simulink model "StateSpace_Sim"  (R2018b)
settings: Solver=ode8  StartTime=0.0  StopTime=30  FixedStep=1/6  RelTol=1e-3
undefined symbols (not defined in the file): A, B, C, d_initial, K, L, M, x_initial, x_lin_i, x_soll
settings Model: Creator=Naresh  LastModifiedBy=Naresh

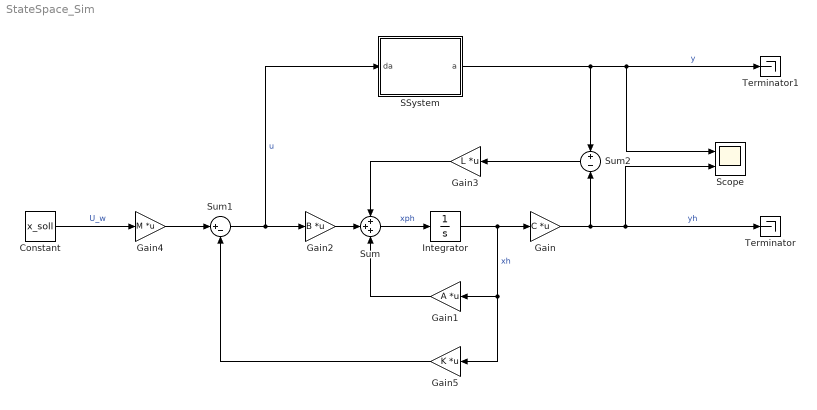
== system StateSpace_Sim ==
  Constant : Constant  Value=x_soll
  Gain : Gain  Gain=C  Multiplication=Matrix(K*u)
  Gain1 : Gain  Gain=A  Multiplication=Matrix(K*u)
  Gain2 : Gain  Gain=B  Multiplication=Matrix(K*u)
  Gain3 : Gain  Gain=L  Multiplication=Matrix(K*u)
  Gain4 : Gain  Gain=M  Multiplication=Matrix(K*u)
  Gain5 : Gain  Gain=K  Multiplication=Matrix(K*u)
  Integrator : Integrator  InitialCondition=x_lin_i
  SSystem : Subsystem
  Scope : Scope  NumInputPorts=2
  Sum : Sum  Inputs=+++
  Sum1 : Sum  Inputs=|+-
  Sum2 : Sum  Inputs=+|-
  Terminator : Terminator
  Terminator1 : Terminator
  wires:
  Integrator/1 -> Gain5/1, Gain1/1, Gain/1  "xh"
  Sum/1 -> Integrator/1  "xph"
  Sum1/1 -> SSystem/1(da), Gain2/1  "u"
  Gain4/1 -> Sum1/1
  Gain/1 -> Terminator/1, Scope/2, Sum2/2  "yh"
  SSystem/1(a) -> Sum2/1, Scope/1, Terminator1/1  "y"
  Sum2/1 -> Gain3/1
  Gain2/1 -> Sum/2
  Gain1/1 -> Sum/3
  Gain3/1 -> Sum/1
  Gain5/1 -> Sum1/2
  Constant/1 -> Gain4/1  "U_w"

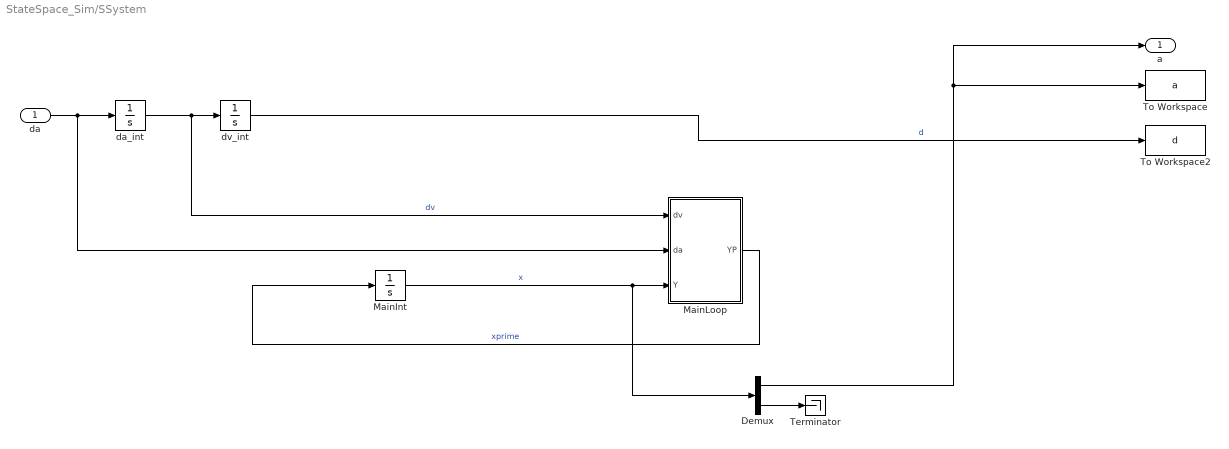
== system StateSpace_Sim/SSystem ==
  da : Inport
  Demux : Demux  Outputs=2
  MainInt : Integrator  InitialCondition=x_initial
  MainLoop : MATLAB Function  TreatAsAtomicUnit=on
  Terminator : Terminator
  To Workspace : ToWorkspace  VariableName=a  SaveFormat=Timeseries  SampleTime=-1
  To Workspace2 : ToWorkspace  VariableName=d  SaveFormat=Timeseries  SampleTime=-1
  da_int : Integrator  InitialCondition=d_initial(2)
  dv_int : Integrator  InitialCondition=d_initial(1)
  a : Outport
  wires:
  da/1 -> MainLoop/2(da), da_int/1
  MainInt/1 -> Demux/1, MainLoop/3(Y)  "x"
  da_int/1 -> MainLoop/1(dv), dv_int/1  "dv"
  MainLoop/1(YP) -> MainInt/1  "xprime"
  dv_int/1 -> To Workspace2/1  "d"
  Demux/2 -> Terminator/1
  Demux/1 -> a/1, To Workspace/1

== matlab function StateSpace_Sim/SSystem/MainLoop ==
  data: dv input; YP output; da input; Y input
function YP = MainLoop(dv,da,Y)
    g = 9.81;
    L = 10;
    m=2;
    lambda=1;

    YP = zeros(2,1);

    YP(1) = Y(2);
    YP(2) = (-L * lambda * Y(2) - dv * cos(Y(1)) * lambda - da * cos(Y(1)) * m - sin(Y(1)) * g * m) / L / m;

end
